simulink model "lift_for_5_floor_building"  (R2020b)
settings: Solver=FixedStepDiscrete  StartTime=0.0  StopTime=10.0  FixedStep=0.1  RelTol=1e-3  EnableMultiTasking=on
settings Model: Creator=user  LastModifiedBy=user
settings SolverCC: AutoInsertRateTranBlk=on
settings DataIOCC: LimitDataPoints=on
settings OptimizationCC: LifeSpan=inf
settings DebuggingCC: AllowSymbolicDim=off  SFUnexpectedBacktrackingDiag=warning  SFNoUnconditionalDefaultTransitionDiag=warning  SFExecutionAtInitializationDiag=none  ArithmeticOperatorsInVariantConditions=warning
settings SFSimCC: SimUseLocalCustomCode=off  CustomCodeUndefinedFunction=UseInterfaceOnly
settings RTWCC: RTWUseLocalCustomCode=off
settings CodeAppCC: StateflowObjectComments=on
settings GRTTargetCC: TargetLangStandard=C89/C90 (ANSI)
settings ConfigComp: CovMetricSettings=dw  CovSaveCumulativeToWorkspaceVar=on  CovSaveSingleToWorkspaceVar=on  CovExternalEMLEnable=off  CovSFcnEnable=off

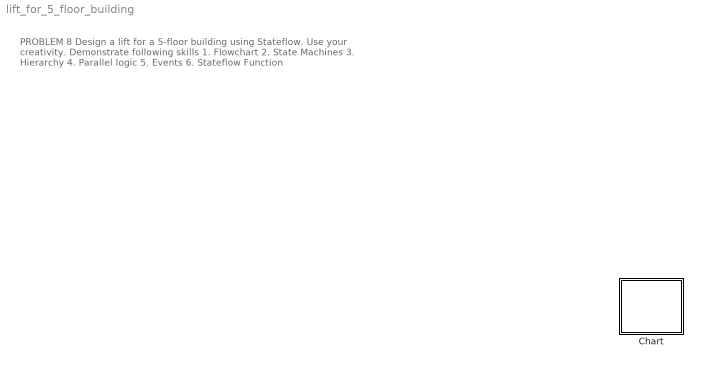
== system lift_for_5_floor_building ==
  note: PROBLEM 8
      |
      | Design a lift for a 5-floor building using Stateflow. Use your creativity. Demonstrate following skills
      | 1. Flowchart
      | 2. State Machines
      | 3. Hierarchy
      | 4. Parallel logic
      | 5. Events
      | 6. Stateflow Function
  Chart : Stateflow chart  TreatAsAtomicUnit=on

== stateflow chart lift_for_5_floor_building/Chart ==
